simulink model "get_data_model"  (R2025b)
settings: Solver=VariableStepAuto  StartTime=0.0  StopTime=10.0  RelTol=1e-3
undefined symbols (not defined in the file or in its folder): STM32_ODR
libraries: etargetslib x11, instrumentseriallib x3
settings Model: Creator=tmood  LastModifiedBy=tmood

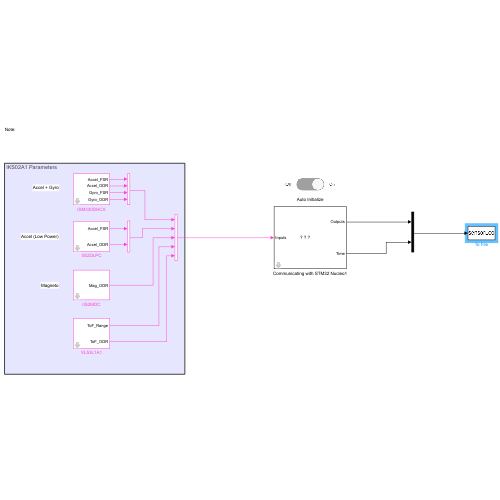
[thumbnail: Simulink's stored preview of the top-level diagram]
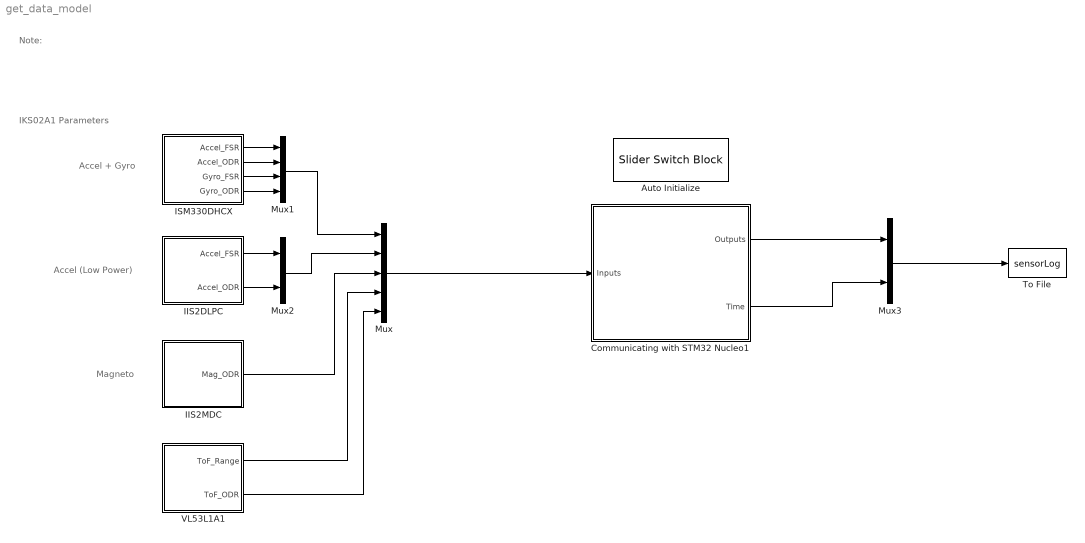
== system get_data_model ==
  note: Accel (Low Power)
  note: Accel + Gyro
  note: Magneto
  note: Note:
  note: IKS02A1 Parameters
  Auto Initialize : SliderSwitchBlock  LabelPosition=Hide
  Communicating with STM32 Nucleo1 : Subsystem  mask{Auto_Initalize=1}
      mask prompts: Auto_Initalize "Automate Initialization?"
      mask TypeOptions Auto_Initalize: 1 | 0
      mask DialogControl Control1 Prompt: Block for communication between host machine and STM32 Nucleo F411RE
      mask Display: image('stm32_icon.png', [0,0,0,0,80,80]);
  IIS2DLPC : Subsystem  mask{FSR_AccelOption=16, ODR_AccelOption=25}
      mask prompts: FSR_AccelOption "Full Scale Range (g)"; ODR_AccelOption "Output Data Rate (Hz)"
      mask init:
      | FSR_AccelVals = [2, 4, 8, 16];
      |     FSR_AccelVal = FSR_AccelVals(FSR_AccelOption);
      |     
      |     ODR_AccelVals = [0 , 1.6 , 12.5 , 25 , 50 , 100 , 200 , 400 , 800 , 1600];
      |     ODR_AccelVal = ODR_AccelVals(ODR_AccelOption);
      mask TypeOptions FSR_AccelOption: 2 | 4 | 8 | 16
      mask TypeOptions ODR_AccelOption: 0 | 1.6 | 12.5 | 25 | 50 | 100 | 200 | 400 | 800 | 1600
      mask DialogControl DescGroupVar Prompt: Accelerometer
  IIS2MDC : Subsystem  mask{ODR_MagOption=20}
      mask prompts: ODR_MagOption "Output Data Rate (Hz)"
      mask init:
      | ODR_MagVals = [10 , 20 , 50 , 100];
      |     ODR_MagVal = ODR_MagVals(ODR_MagOption);
      mask TypeOptions ODR_MagOption: 10 | 20 | 50 | 100
      mask DialogControl DescGroupVar Prompt: Magnetometer
  ISM330DHCX : Subsystem  mask{FSR_AccelOption=16, ODR_AccelOption=52, FSR_GyroOption=4000, ODR_GyroOption=52}
      mask prompts: FSR_AccelOption "Full Scale Range (g)"; ODR_AccelOption "Output Data Rate (Hz)"; FSR_GyroOption "Full Scale Range (dps)"; ODR_GyroOption "Output Data Rate (Hz)"
      mask init:
      | FSR_AccelVals = [2, 4, 8, 16];
      |     FSR_AccelVal = FSR_AccelVals(FSR_AccelOption);
      |     
      |     ODR_AccelVals = [0 , 12.5 , 16 , 52 , 104 , 208 , 416 , 833 , 1666 , 3332 , 6667];
      |     ODR_AccelVal = ODR_AccelVals(ODR_AccelOption);
      | 
      |     FSR_GyroVals = [125, 250, 500, 1000, 2000, 4000];
      |     FSR_GyroVal = FSR_GyroVals(FSR_GyroOption);
      | 
      |     ODR_GyroVals = [0 , 12.5 , 16 , 52 , 104 , 208 , 416 , 833 , 1666 , 3332 , 6667];
      |     ODR_GyroVal = ODR_GyroVals(ODR_GyroOption);
      mask TypeOptions FSR_AccelOption: 2 | 4 | 8 | 16
      mask TypeOptions ODR_AccelOption: 0 | 12.5 | 16 | 52 | 104 | 208 | 416 | 833 | 1666 | 3332 | 6667
      mask TypeOptions FSR_GyroOption: 125 | 250 | 500 | 1000 | 2000 | 4000
      mask TypeOptions ODR_GyroOption: 0 | 12.5 | 16 | 52 | 104 | 208 | 416 | 833 | 1666 | 3332 | 6667
      mask DialogControl DescGroupVar Prompt: Accelerometer
      mask DialogControl DescGroupVar_copy Prompt: Gyroscope
  Mux : Mux  Inputs=5
  Mux1 : Mux
  Mux2 : Mux  Inputs=2
  Mux3 : Mux  Inputs=2
  To File : ToFile  Filename=sensorLog  MatrixName=LogData
  VL53L1A1 : Subsystem  mask{FSR_TOFOption=Short, ODR_TOFOption=10}
      mask prompts: FSR_TOFOption "Ranging Profile"; ODR_TOFOption "Output Data Rate (Hz)"
      mask init:
      | FSR_TOFVals = [1 , 2];
      |     FSR_TOF = FSR_TOFVals(FSR_TOFOption);
      |     
      |     ODR_TOFVals = [1 , 5, 10, 20, 30];
      |     ODR_TOF = ODR_TOFVals(ODR_TOFOption);
      mask TypeOptions FSR_TOFOption: Short | Long
      mask TypeOptions ODR_TOFOption: 1 | 5 | 10 | 20 | 30
      mask DialogControl DescGroupVar Prompt: Time of Flight Sensor 1x3
  wires:
  IIS2MDC/1(Mag_ODR) -> Mux/3
  IIS2DLPC/1(Accel_FSR) -> Mux2/1
  ISM330DHCX/3(Gyro_FSR) -> Mux1/3
  Mux2/1 -> Mux/2
  Mux1/1 -> Mux/1
  ISM330DHCX/2(Accel_ODR) -> Mux1/2
  Mux/1 -> Communicating with STM32 Nucleo1/1(Inputs)
  IIS2DLPC/2(Accel_ODR) -> Mux2/2
  ISM330DHCX/4(Gyro_ODR) -> Mux1/4
  ISM330DHCX/1(Accel_FSR) -> Mux1/1
  VL53L1A1/1(ToF_Range) -> Mux/4
  VL53L1A1/2(ToF_ODR) -> Mux/5
  Communicating with STM32 Nucleo1/1(Outputs) -> Mux3/1
  Communicating with STM32 Nucleo1/2(Time) -> Mux3/2
  Mux3/1 -> To File/1

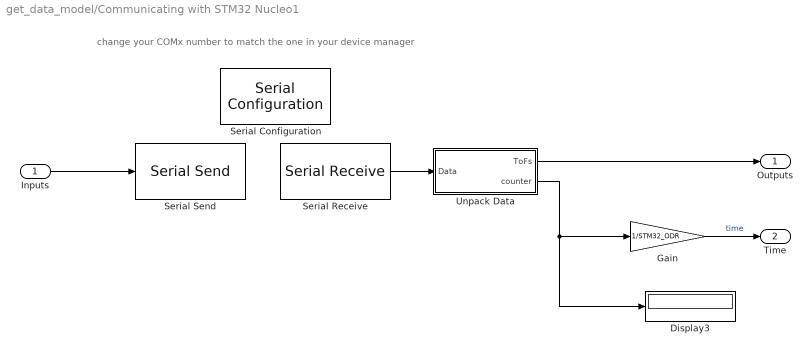
== system get_data_model/Communicating with STM32 Nucleo1 ==
  note: change your COMx number to match the one in your device manager
  Inputs : Inport
  Display3 : Display
  Gain : Gain  Gain=1/STM32_ODR
  Serial Configuration : instrumentseriallib/Serial Configuration  Priority=-200000  PortSel=STLINK_COMPORT  Port=STLINK_COMPORT  ComPort=STLINK_COMPORT  BaudRate=1843200  DataBits=8  Parity=even  StopBits=2  ByteOrder=little-endian  FlowControl=none  Timeout=5  SimulateUsing=Interpreted execution  BlockInModel=on  aMode=1
      settings: LibrarySourceBlock=embeddedtargetslib/Host Communication/Serial Configuration
  Serial Receive : instrumentseriallib/Serial Receive  Priority=1  PortSel=STLINK_COMPORT  Port=STLINK_COMPORT  ComPort=STLINK_COMPORT  DataType=single  SaveDataType=uint8  ToggleHeader=on  Header='J_A'  ToggleDataSize=on  DataSize=[1 4*3+1]  ToggleTerminator=on  Terminator=Custom terminator  CustomTerminator='A_J'  InputFormat=Column major  EnableBlockingMode=on  ActionDataUnavailable=Output last received value  ActionWhenDataUnavailable=Output last received value  CustomValue=0  SampleTime=1/STM32_ODR  SimulateUsing=Interpreted execution  BlockInModel=on  aMode=1
      settings: LibrarySourceBlock=embeddedtargetslib/Host Communication/Serial Receive
  Serial Send : instrumentseriallib/Serial Send  Priority=1  PortSel=STLINK_COMPORT  Port=STLINK_COMPORT  ComPort=STLINK_COMPORT  Header='J_A'  Terminator=Custom terminator  CustomTerminator='A_J'  EnableBlockingMode=off  SimulateUsing=Interpreted execution  BlockInModel=on  aMode=1
      settings: LibrarySourceBlock=embeddedtargetslib/Host Communication/Serial Send
  Unpack Data : Subsystem
  Outputs : Outport
  Time : Outport  Port=2
  wires:
  Unpack Data/2(counter) -> Display3/1, Gain/1
  Gain/1 -> Time/1  "time"
  Unpack Data/1(ToFs) -> Outputs/1
  Serial Receive/1 -> Unpack Data/1(Data)
  Inputs/1 -> Serial Send/1

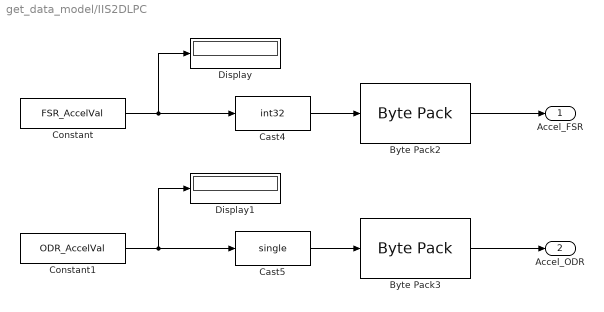
== system get_data_model/IIS2DLPC ==
  Byte Pack2 : etargetslib/Byte Pack  datatypes={'int32'}  byteAlign=1
  Byte Pack3 : etargetslib/Byte Pack  datatypes={'single'}  byteAlign=1
  Cast4 : DataTypeConversion  OutDataTypeStr=int32  SaturateOnIntegerOverflow=off  RndMeth=Floor
  Cast5 : DataTypeConversion  OutDataTypeStr=single  SaturateOnIntegerOverflow=off  RndMeth=Floor
  Constant : Constant  Value=FSR_AccelVal
  Constant1 : Constant  Value=ODR_AccelVal
  Display : Display
  Display1 : Display
  Accel_FSR : Outport
  Accel_ODR : Outport  Port=2
  wires:
  Constant/1 -> Cast4/1, Display/1
  Constant1/1 -> Cast5/1, Display1/1
  Cast4/1 -> Byte Pack2/1
  Cast5/1 -> Byte Pack3/1
  Byte Pack2/1 -> Accel_FSR/1
  Byte Pack3/1 -> Accel_ODR/1

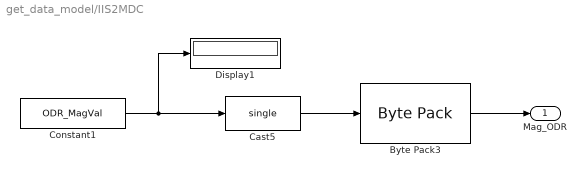
== system get_data_model/IIS2MDC ==
  Byte Pack3 : etargetslib/Byte Pack  datatypes={'single'}  byteAlign=1
  Cast5 : DataTypeConversion  OutDataTypeStr=single  SaturateOnIntegerOverflow=off  RndMeth=Floor
  Constant1 : Constant  Value=ODR_MagVal
  Display1 : Display
  Mag_ODR : Outport
  wires:
  Constant1/1 -> Cast5/1, Display1/1
  Cast5/1 -> Byte Pack3/1
  Byte Pack3/1 -> Mag_ODR/1

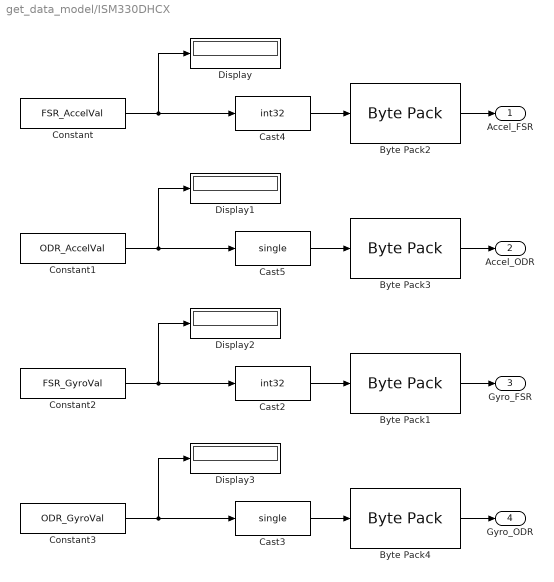
== system get_data_model/ISM330DHCX ==
  Byte Pack1 : etargetslib/Byte Pack  datatypes={'int32'}  byteAlign=1
  Byte Pack2 : etargetslib/Byte Pack  datatypes={'int32'}  byteAlign=1
  Byte Pack3 : etargetslib/Byte Pack  datatypes={'single'}  byteAlign=1
  Byte Pack4 : etargetslib/Byte Pack  datatypes={'single'}  byteAlign=1
  Cast2 : DataTypeConversion  OutDataTypeStr=int32  SaturateOnIntegerOverflow=off  RndMeth=Floor
  Cast3 : DataTypeConversion  OutDataTypeStr=single  SaturateOnIntegerOverflow=off  RndMeth=Floor
  Cast4 : DataTypeConversion  OutDataTypeStr=int32  SaturateOnIntegerOverflow=off  RndMeth=Floor
  Cast5 : DataTypeConversion  OutDataTypeStr=single  SaturateOnIntegerOverflow=off  RndMeth=Floor
  Constant : Constant  Value=FSR_AccelVal
  Constant1 : Constant  Value=ODR_AccelVal
  Constant2 : Constant  Value=FSR_GyroVal
  Constant3 : Constant  Value=ODR_GyroVal
  Display{,1..3} (4 alike) : Display
  Accel_FSR : Outport
  Accel_ODR : Outport  Port=2
  Gyro_FSR : Outport  Port=3
  Gyro_ODR : Outport  Port=4
  wires:
  Constant/1 -> Cast4/1, Display/1
  Constant1/1 -> Cast5/1, Display1/1
  Constant2/1 -> Cast2/1, Display2/1
  Constant3/1 -> Cast3/1, Display3/1
  Cast4/1 -> Byte Pack2/1
  Cast5/1 -> Byte Pack3/1
  Cast2/1 -> Byte Pack1/1
  Cast3/1 -> Byte Pack4/1
  Byte Pack2/1 -> Accel_FSR/1
  Byte Pack3/1 -> Accel_ODR/1
  Byte Pack1/1 -> Gyro_FSR/1
  Byte Pack4/1 -> Gyro_ODR/1

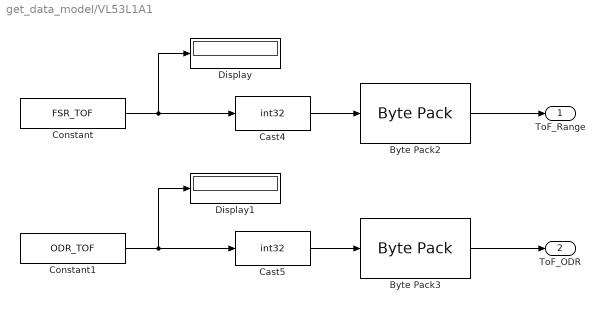
== system get_data_model/VL53L1A1 ==
  Byte Pack2 : etargetslib/Byte Pack  datatypes={'int32'}  byteAlign=1
  Byte Pack3 : etargetslib/Byte Pack  datatypes={'int32'}  byteAlign=1
  Cast4 : DataTypeConversion  OutDataTypeStr=int32  SaturateOnIntegerOverflow=off  RndMeth=Floor
  Cast5 : DataTypeConversion  OutDataTypeStr=int32  SaturateOnIntegerOverflow=off  RndMeth=Floor
  Constant : Constant  Value=FSR_TOF
  Constant1 : Constant  Value=ODR_TOF
  Display : Display
  Display1 : Display
  ToF_Range : Outport
  ToF_ODR : Outport  Port=2
  wires:
  Constant/1 -> Cast4/1, Display/1
  Constant1/1 -> Cast5/1, Display1/1
  Cast4/1 -> Byte Pack2/1
  Cast5/1 -> Byte Pack3/1
  Byte Pack2/1 -> ToF_Range/1
  Byte Pack3/1 -> ToF_ODR/1

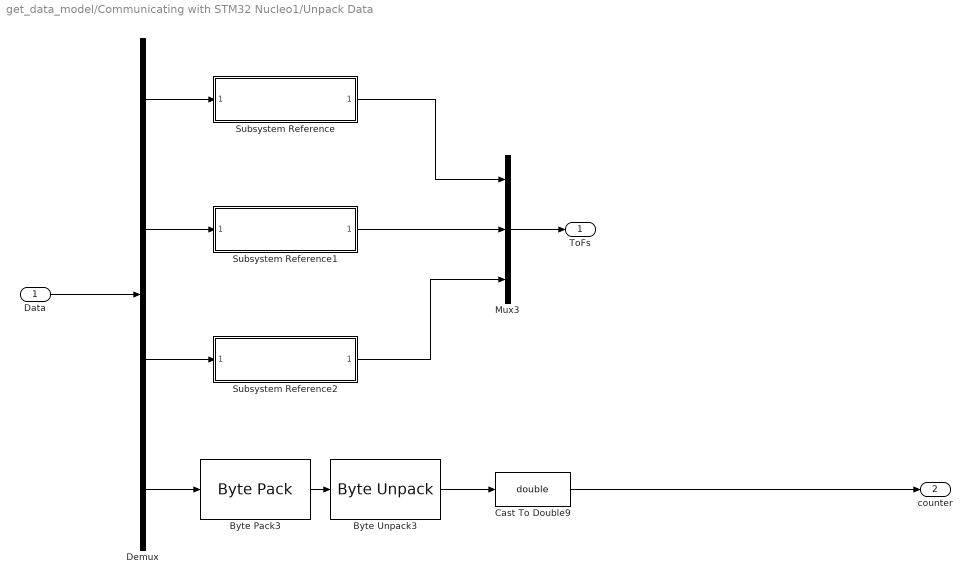
== system get_data_model/Communicating with STM32 Nucleo1/Unpack Data ==
  Data : Inport
  Byte Pack3 : etargetslib/Byte Pack  datatypes={'single'}  byteAlign=1
  Byte Unpack3 : etargetslib/Byte Unpack  dimensions={[1]}  datatypes={'uint32'}  byteAlign=1
      settings: LibrarySourceBlock=embeddedtargetslib/Host Communication/Byte Unpack
  Cast To Double9 : DataTypeConversion  OutDataTypeStr=double  SaturateOnIntegerOverflow=off  RndMeth=Floor
  Demux : Demux  Outputs=[4 4 4 1]
  Mux3 : Mux  Inputs=[4 4 4]
  Subsystem Reference : Subsystem  ReferencedSubsystem=unpack_ToF
  Subsystem Reference1 : Subsystem  ReferencedSubsystem=unpack_ToF
  Subsystem Reference2 : Subsystem  ReferencedSubsystem=unpack_ToF
  ToFs : Outport
  counter : Outport  Port=2
  wires:
  Mux3/1 -> ToFs/1
  Data/1 -> Demux/1
  Cast To Double9/1 -> counter/1
  Byte Unpack3/1 -> Cast To Double9/1
  Byte Pack3/1 -> Byte Unpack3/1
  Demux/4 -> Byte Pack3/1
  Demux/1 -> Subsystem Reference/1
  Demux/2 -> Subsystem Reference1/1
  Demux/3 -> Subsystem Reference2/1
  Subsystem Reference/1 -> Mux3/1
  Subsystem Reference1/1 -> Mux3/2
  Subsystem Reference2/1 -> Mux3/3
